simulink model "StartStop"  (R2021a)
settings: Solver=VariableStepAuto  StartTime=0.0  StopTime=10.0  RelTol=1e-3
undefined symbols (not defined in the file): cs_charge_deplete_bool, cs_electric_decel_spd, cs_electric_launch_spd_hi, cs_electric_launch_spd_lo, cs_hi_soc, cs_lo_soc, cs_off_trq_frac, cyc_mph, fc_map_spd, fc_max_trq, fc_on, fc_spd_scale, fc_trq_scale, fc_tstat, mc_map_spd, mc_max_trq, mc_overtrq_factor, mc_spd_scale, mc_trq_scale, tc_mc_to_fc_ratio, vc_fc_warm_tmp_frac, vc_idle_bool, vc_idle_spd, vc_key_on, vc_launch_spd
settings Model: Creator=thyag  LastModifiedBy=thyag

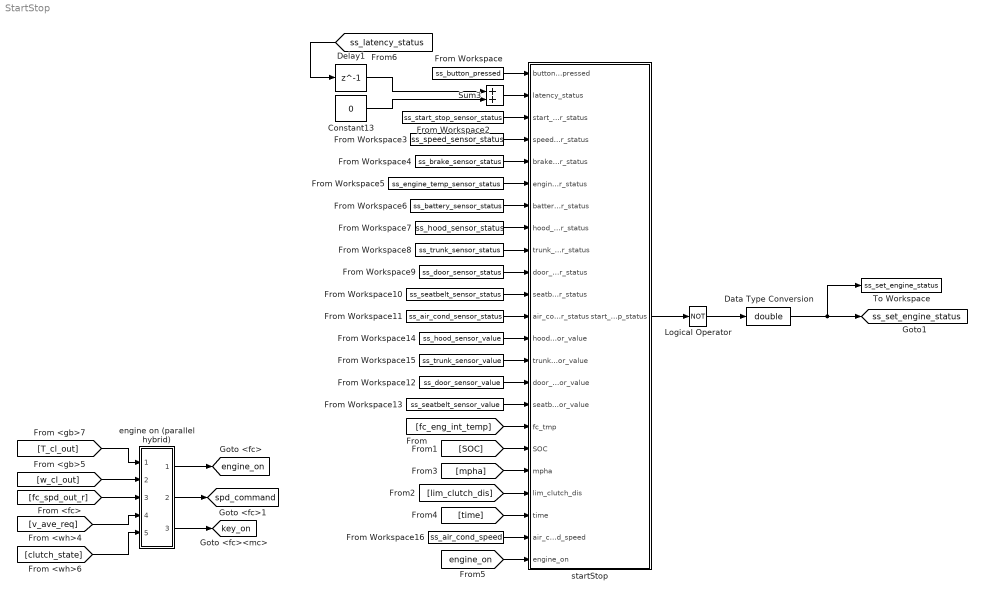
== system StartStop ==
  Constant13 : Constant  Value=0  OutDataTypeStr=fixdt(0,1,1,0)
  Data Type Conversion : DataTypeConversion  OutDataTypeStr=double
  Delay1 : Delay  DelayLength=1  InitialCondition=0
  From Workspace : FromWorkspace  VariableName=ss_button_pressed
  From Workspace10 : FromWorkspace  VariableName=ss_seatbelt_sensor_status
  From Workspace11 : FromWorkspace  VariableName=ss_air_cond_sensor_status
  From Workspace12 : FromWorkspace  VariableName=ss_door_sensor_value
  From Workspace13 : FromWorkspace  VariableName=ss_seatbelt_sensor_value
  From Workspace14 : FromWorkspace  VariableName=ss_hood_sensor_value
  From Workspace15 : FromWorkspace  VariableName=ss_trunk_sensor_value
  From Workspace16 : FromWorkspace  VariableName=ss_air_cond_speed
  From Workspace2 : FromWorkspace  VariableName=ss_start_stop_sensor_status
  From Workspace3 : FromWorkspace  VariableName=ss_speed_sensor_status
  From Workspace4 : FromWorkspace  VariableName=ss_brake_sensor_status
  From Workspace5 : FromWorkspace  VariableName=ss_engine_temp_sensor_status
  From Workspace6 : FromWorkspace  VariableName=ss_battery_sensor_status
  From Workspace7 : FromWorkspace  VariableName=ss_hood_sensor_status
  From Workspace8 : FromWorkspace  VariableName=ss_trunk_sensor_status
  From Workspace9 : FromWorkspace  VariableName=ss_door_sensor_status
  Logical Operator : Logic  Operator=NOT  AllPortsSameDT=off  OutDataTypeStr=fixdt(0,1,1,0)
  Sum3 : Sum  OutDataTypeStr=fixdt(0,1,1,0)
  To Workspace : ToWorkspace  VariableName=ss_set_engine_status  SampleTime=1
  engine on (parallel hybrid) : Subsystem
  startStop : Subsystem
  tag scope: engine_on=global, key_on=global, spd_command=global, ss_set_engine_status=global
  wires:
  engine on (parallel hybrid)/2(spd command (rad/s)) -> [spd_command]
  [v_ave_req] -> engine on (parallel hybrid)/4(v_ave_req)
  [ss_latency_status] -> Delay1/1
  [time] -> startStop/21(time)
  [engine_on] -> startStop/23(engine_on)
  Sum3/1 -> startStop/2(latency_status)
  Data Type Conversion/1 -> [ss_set_engine_status], To Workspace/1
  From Workspace13/1 -> startStop/16(seatbelt_sensor_value)
  From Workspace2/1 -> startStop/3(start_stop_sensor_status)
  Delay1/1 -> Sum3/1
  Constant13/1 -> Sum3/2
  From Workspace6/1 -> startStop/7(battery_sensor_status)
  From Workspace14/1 -> startStop/13(hood_sensor_value)
  From Workspace/1 -> startStop/1(button_pressed)
  [w_cl_out] -> engine on (parallel hybrid)/2(spd req'd out of clutch (N*m)1)
  [clutch_state] -> engine on (parallel hybrid)/5(clutch state)
  From Workspace8/1 -> startStop/9(trunk_sensor_status)
  startStop/1(start_stop_status) -> Logical Operator/1
  [T_cl_out] -> engine on (parallel hybrid)/1(trq req'd out of clutch (N*m))
  engine on (parallel hybrid)/3(key on) -> [key_on]
  [SOC] -> startStop/18(SOC)
  [fc_eng_int_temp] -> startStop/17(fc_tmp)
  [fc_spd_out_r] -> engine on (parallel hybrid)/3(fc_spd_out_r)
  From Workspace7/1 -> startStop/8(hood_sensor_status)
  Logical Operator/1 -> Data Type Conversion/1
  From Workspace15/1 -> startStop/14(trunk_sensor_value)
  From Workspace3/1 -> startStop/4(speed_sensor_status)
  From Workspace9/1 -> startStop/10(door_sensor_status)
  [mpha] -> startStop/19(mpha)
  engine on (parallel hybrid)/1(engine on) -> [engine_on]
  From Workspace12/1 -> startStop/15(door_sensor_value)
  From Workspace11/1 -> startStop/12(air_cond_sensor_status)
  From Workspace5/1 -> startStop/6(engine_temp_sensor_status)
  From Workspace10/1 -> startStop/11(seatbelt_sensor_status)
  [lim_clutch_dis] -> startStop/20(lim_clutch_dis)
  From Workspace16/1 -> startStop/22(air_cond_speed)
  From Workspace4/1 -> startStop/5(brake_sensor_status)

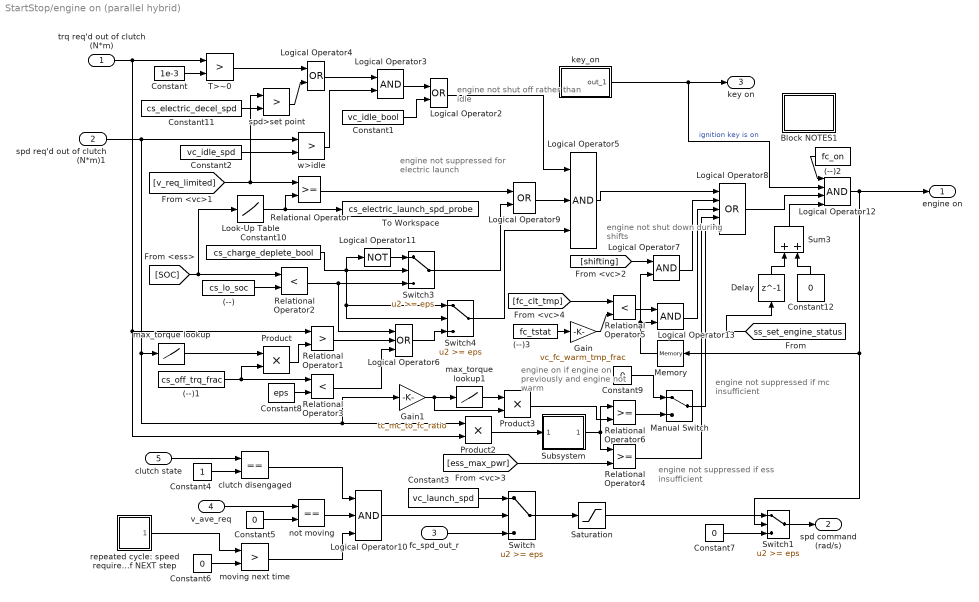
== system StartStop/engine on (parallel hybrid) ==
  note: engine not suppressed
      | if mc insufficient
  note: engine not shut
      | down during shifts
  note: engine on if engine on
      | previously and engine
      | not warm
  note: engine not shut off
      |  rather than idle
  note: engine not
      | suppressed for
      | electric launch
  note: engine not suppressed if
      | ess insufficient
  trq req'd out of clutch (N*m) : Inport
  spd req'd out of clutch (N*m)1 : Inport  Port=2
  fc_spd_out_r : Inport  Port=3
  v_ave_req : Inport  Port=4
  clutch state : Inport  Port=5
  (--) : Constant  Value=cs_lo_soc
  (--)1 : Constant  Value=cs_off_trq_frac
  (--)2 : Constant  Value=fc_on
  (--)3 : Constant  Value=fc_tstat
  Block NOTES1 : Subsystem
      mask Display: disp('Block\nNOTES')
  Constant : Constant  Value=1e-3
  Constant1 : Constant  Value=vc_idle_bool
  Constant10 : Constant  Value=cs_charge_deplete_bool
  Constant11 : Constant  Value=cs_electric_decel_spd
  Constant{5..7,9,12} (5 alike) : Constant  Value=0
  Constant2 : Constant  Value=vc_idle_spd
  Constant3 : Constant  Value=vc_launch_spd
  Constant4 : Constant
  Constant8 : Constant  Value=eps
  Delay : Delay  DelayLength=1  InitialCondition=1
  Gain : Gain  Gain=vc_fc_warm_tmp_frac  SaturateOnIntegerOverflow=on  OutDataTypeStr=Inherit: Same as input  ParamDataTypeStr=Inherit: Same as input
  Gain1 : Gain  Gain=tc_mc_to_fc_ratio  SaturateOnIntegerOverflow=on  OutDataTypeStr=Inherit: Same as input  ParamDataTypeStr=Inherit: Same as input
  Logical Operator10 : Logic  Inputs=3
  Logical Operator11 : Logic  Operator=NOT  Inputs=1
  Logical Operator12 : Logic  Inputs=4
  Logical Operator13 : Logic
  Logical Operator2 : Logic  Operator=OR
  Logical Operator3 : Logic
  Logical Operator4 : Logic  Operator=OR
  Logical Operator5 : Logic  Inputs=3
  Logical Operator6 : Logic  Operator=OR  Inputs=3
  Logical Operator7 : Logic
  Logical Operator8 : Logic  Operator=OR  Inputs=5
  Logical Operator9 : Logic  Operator=OR
  Look-Up Table : Lookup  InputValues=[cs_lo_soc cs_hi_soc cs_hi_soc+eps]  Table=[cs_electric_launch_spd_lo cs_electric_launch_spd_hi cs_electric_launch_spd_hi]  SaturateOnIntegerOverflow=on
  Manual Switch : ManualSwitch
  Memory : Memory  InitialCondition=cyc_mph(1,2)>0
  Product : Product  InputSameDT=on  RndMeth=Zero  SaturateOnIntegerOverflow=on  OutDataTypeStr=Inherit: Same as first input
  Product2 : Product  InputSameDT=on  RndMeth=Zero  SaturateOnIntegerOverflow=on  OutDataTypeStr=Inherit: Same as first input
  Product3 : Product  InputSameDT=on  RndMeth=Zero  SaturateOnIntegerOverflow=on  OutDataTypeStr=Inherit: Same as first input
  Relational Operator : RelationalOperator  RndMeth=Nearest  InputSameDT=on
  Relational Operator1 : RelationalOperator  Operator=>  RndMeth=Nearest  InputSameDT=on
  Relational Operator2 : RelationalOperator  Operator=<  RndMeth=Nearest  InputSameDT=on
  Relational Operator3 : RelationalOperator  Operator=<  RndMeth=Nearest  InputSameDT=on
  Relational Operator4 : RelationalOperator  RndMeth=Nearest  InputSameDT=on
  Relational Operator5 : RelationalOperator  Operator=<  RndMeth=Nearest  InputSameDT=on
  Relational Operator6 : RelationalOperator  RndMeth=Nearest  InputSameDT=on
  Saturation : Saturate  UpperLimit=max(fc_map_spd)*fc_spd_scale  LowerLimit=vc_idle_spd*vc_idle_bool
  Subsystem : Subsystem  mask(Running Average){n=3}
      mask prompts: n "Averaging Time Steps (#)"
      mask help: Running Average
      mask Help: Output is the average of the last (Averaging Time) seconds of input.
      mask Display: disp('Running\nAverage')
  Sum3 : Sum  Inputs=+|+
  Switch{,1,3..4} (4 alike) : Switch  Threshold=eps  SaturateOnIntegerOverflow=on  InputSameDT=on
  T>~0 : RelationalOperator  Operator=>  RndMeth=Nearest  InputSameDT=on
  To Workspace : ToWorkspace  VariableName=cs_electric_launch_spd_probe  SampleTime=-1
  clutch disengaged : RelationalOperator  Operator===  RndMeth=Nearest  InputSameDT=on
  key_on : Subsystem  mask(Repeating table){t=vc_key_on(:,1), y=vc_key_on(:,2)}
      mask prompts: t "Time values:"; y "Output values:"
      mask help:
      | Repeating table.
      | Enter values of time and output for first cycle.
      mask init:
      | period = max(t);
      mask Help: Repeats cycle given in table. Time values should be monotonically increasing.
  max_torque lookup : Lookup  InputValues=fc_map_spd*fc_spd_scale  Table=fc_max_trq*fc_trq_scale  SaturateOnIntegerOverflow=on
  max_torque lookup1 : Lookup  InputValues=mc_map_spd*mc_spd_scale  Table=mc_max_trq*mc_trq_scale*mc_overtrq_factor  SaturateOnIntegerOverflow=on
  moving next time : RelationalOperator  Operator=>  RndMeth=Nearest  InputSameDT=on
  not moving : RelationalOperator  Operator===  RndMeth=Nearest  InputSameDT=on
  repeated cycle: speed required at end of NEXT step : Subsystem  mask(Forward looking repeating table){t=cyc_mph(:,1), y=cyc_mph(:,2)}
      mask prompts: t "Time values:"; y "Output values:"
      mask help:
      | Forward looking repeating table.
      | Enter values of time and output for first cycle.
      mask init:
      | period = max(t);
      mask Help: Repeats cycle given in table with a one time step forward offset. Time values should be monotonically increasing.
  spd>set point : RelationalOperator  Operator=>  RndMeth=Nearest  InputSameDT=on
  w>idle : RelationalOperator  Operator=>  RndMeth=Nearest  InputSameDT=on
  engine on : Outport
  spd command (rad/s) : Outport  Port=2
  key on : Outport  Port=3
  wires:
  Subsystem/1(out_1) -> Relational Operator6/1, Relational Operator4/1
  Product3/1 -> Relational Operator6/2
  [ess_max_pwr] -> Relational Operator4/2
  [v_req_limited] -> spd>set point/1, Relational Operator/1
  T>~0/1 -> Logical Operator4/1
  Logical Operator4/1 -> Logical Operator3/1
  spd>set point/1 -> Logical Operator4/2
  Constant11/1 -> spd>set point/2
  spd req'd out of clutch (N*m)1/1 -> w>idle/1, Gain1/1, Product2/1, max_torque lookup/1
  w>idle/1 -> Logical Operator3/2
  Constant2/1 -> w>idle/2
  Constant9/1 -> Manual Switch/1
  Manual Switch/1 -> Logical Operator8/5
  Relational Operator6/1 -> Manual Switch/2
  Gain1/1 -> Product3/2, max_torque lookup1/1
  max_torque lookup1/1 -> Product3/1
  Relational Operator3/1 -> Logical Operator6/3
  Product2/1 -> Subsystem/1(in_1)
  Constant4/1 -> clutch disengaged/2
  clutch state/1 -> clutch disengaged/1
  Constant5/1 -> not moving/2
  v_ave_req/1 -> not moving/1
  not moving/1 -> Logical Operator10/2
  moving next time/1 -> Logical Operator10/3
  clutch disengaged/1 -> Logical Operator10/1
  Constant6/1 -> moving next time/2
  repeated cycle: speed required at end of NEXT step/1(out_1) -> moving next time/1
  Constant7/1 -> Switch1/3
  Switch1/1 -> spd command (rad/s)/1
  Saturation/1 -> Switch1/1
  fc_spd_out_r/1 -> Switch/3
  Logical Operator10/1 -> Switch/2
  Switch/1 -> Saturation/1
  Constant3/1 -> Switch/1
  Relational Operator4/1 -> Logical Operator8/4
  (--)/1 -> Relational Operator2/2
  [SOC] -> Look-Up Table/1, Relational Operator2/1
  Logical Operator11/1 -> Switch3/1
  Relational Operator2/1 -> Logical Operator6/1, Switch3/3
  Constant10/1 -> Logical Operator11/1, Switch3/2, Switch4/2, Switch4/1
  Look-Up Table/1 -> To Workspace/1, Relational Operator/2
  Relational Operator/1 -> Logical Operator9/1
  Switch4/1 -> Logical Operator5/3
  Logical Operator9/1 -> Logical Operator5/2
  Logical Operator2/1 -> Logical Operator5/1
  key_on/1(out_1) -> Logical Operator12/2, key on/1  "ignition key is on"
  Logical Operator8/1 -> Logical Operator12/3
  (--)3/1 -> Gain/1
  Gain/1 -> Relational Operator5/2
  Logical Operator13/1 -> Logical Operator8/3
  [fc_clt_tmp] -> Relational Operator5/1
  Relational Operator5/1 -> Logical Operator13/1
  Memory/1 -> Logical Operator13/2, Logical Operator7/2
  Relational Operator1/1 -> Logical Operator6/2
  Logical Operator5/1 -> Logical Operator8/1
  Logical Operator3/1 -> Logical Operator2/1
  Constant1/1 -> Logical Operator2/2
  trq req'd out of clutch (N*m)/1 -> Relational Operator1/1, Product2/2, T>~0/1
  Logical Operator7/1 -> Logical Operator8/2
  [shifting] -> Logical Operator7/1
  Constant/1 -> T>~0/2
  Switch3/1 -> Logical Operator9/2
  Logical Operator6/1 -> Switch4/3
  Constant8/1 -> Relational Operator3/2
  (--)1/1 -> Relational Operator3/1, Product/2
  Product/1 -> Relational Operator1/2
  max_torque lookup/1 -> Product/1
  (--)2/1 -> Logical Operator12/1
  Logical Operator12/1 -> engine on/1, Memory/1, Switch1/2
  [ss_set_engine_status] -> Delay/1
  Constant12/1 -> Sum3/2
  Sum3/1 -> Logical Operator12/4
  Delay/1 -> Sum3/1

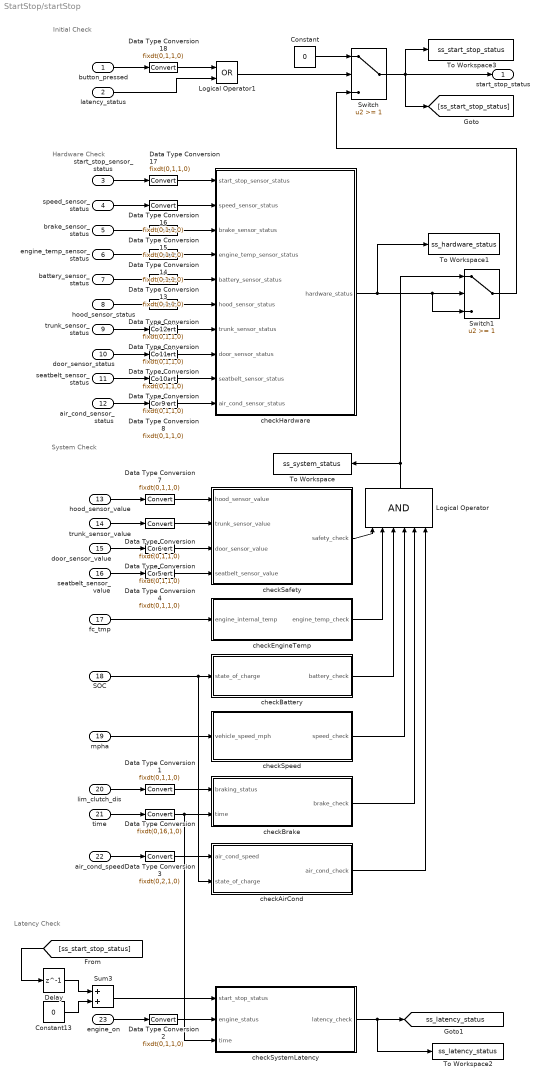
== system StartStop/startStop ==
  note: Initial Check
  note: Hardware Check
  note: Latency Check
  note: System Check
  button_pressed : Inport
  latency_status : Inport  Port=2
  start_stop_sensor_status : Inport  Port=3
  speed_sensor_status : Inport  Port=4
  brake_sensor_status : Inport  Port=5
  engine_temp_sensor_status : Inport  Port=6
  battery_sensor_status : Inport  Port=7
  hood_sensor_status : Inport  Port=8
  trunk_sensor_status : Inport  Port=9
  door_sensor_status : Inport  Port=10
  seatbelt_sensor_status : Inport  Port=11
  air_cond_sensor_status : Inport  Port=12
  hood_sensor_value : Inport  Port=13
  trunk_sensor_value : Inport  Port=14
  door_sensor_value : Inport  Port=15
  seatbelt_sensor_value : Inport  Port=16
  fc_tmp : Inport  Port=17
  SOC : Inport  Port=18
  mpha : Inport  Port=19
  lim_clutch_dis : Inport  Port=20
  time : Inport  Port=21
  air_cond_speed : Inport  Port=22
  engine_on : Inport  Port=23
  Constant : Constant  Value=0  OutDataTypeStr=fixdt(0,1,1,0)
  Constant13 : Constant  Value=0  OutDataTypeStr=fixdt(0,1,1,0)
  Data Type Conversion : DataTypeConversion  OutDataTypeStr=fixdt(0,16,1,0)
  Data Type Conversion{1..2,4..18} (17 alike) : DataTypeConversion  OutDataTypeStr=fixdt(0,1,1,0)
  Data Type Conversion3 : DataTypeConversion  OutDataTypeStr=fixdt(0,2,1,0)
  Delay : Delay  DelayLength=1  InitialCondition=0
  Logical Operator : Logic  Inputs=6  AllPortsSameDT=off  OutDataTypeStr=fixdt(0,1,1,0)
  Logical Operator1 : Logic  Operator=OR  AllPortsSameDT=off  OutDataTypeStr=fixdt(0,1,1,0)
  Sum3 : Sum  OutDataTypeStr=fixdt(0,1,1,0)
  Switch : Switch  Threshold=1  OutDataTypeStr=fixdt(0,1,1,0)
  Switch1 : Switch  Threshold=1  OutDataTypeStr=fixdt(0,1,1,0)
  To Workspace : ToWorkspace  VariableName=ss_system_status  SampleTime=-1
  To Workspace1 : ToWorkspace  VariableName=ss_hardware_status  SampleTime=-1
  To Workspace2 : ToWorkspace  VariableName=ss_latency_status  SampleTime=-1
  To Workspace3 : ToWorkspace  VariableName=ss_start_stop_status  SampleTime=-1
  checkAirCond : Subsystem
  checkBattery : Subsystem
  checkBrake : Subsystem
  checkEngineTemp : Subsystem
  checkHardware : Subsystem
  checkSafety : Subsystem
  checkSpeed : Subsystem
  checkSystemLatency : Subsystem
  start_stop_status : Outport
  tag scope: ss_latency_status=global
  wires:
  engine_temp_sensor_status/1 -> Data Type Conversion14/1
  speed_sensor_status/1 -> Data Type Conversion16/1
  Switch/1 -> [ss_start_stop_status], start_stop_status/1, To Workspace3/1
  trunk_sensor_status/1 -> Data Type Conversion11/1
  hood_sensor_status/1 -> Data Type Conversion12/1
  brake_sensor_status/1 -> Data Type Conversion15/1
  battery_sensor_status/1 -> Data Type Conversion13/1
  door_sensor_status/1 -> Data Type Conversion10/1
  seatbelt_sensor_status/1 -> Data Type Conversion9/1
  air_cond_sensor_status/1 -> Data Type Conversion8/1
  button_pressed/1 -> Data Type Conversion18/1
  latency_status/1 -> Logical Operator1/2
  Logical Operator1/1 -> Switch/2
  start_stop_sensor_status/1 -> Data Type Conversion17/1
  checkHardware/1(hardware_status) -> Switch1/2, Switch1/3, To Workspace1/1
  hood_sensor_value/1 -> Data Type Conversion7/1
  trunk_sensor_value/1 -> Data Type Conversion6/1
  door_sensor_value/1 -> Data Type Conversion5/1
  seatbelt_sensor_value/1 -> Data Type Conversion4/1
  fc_tmp/1 -> checkEngineTemp/1(engine_internal_temp)
  SOC/1 -> checkAirCond/2(state_of_charge), checkBattery/1(state_of_charge)
  mpha/1 -> checkSpeed/1(vehicle_speed_mph)
  air_cond_speed/1 -> Data Type Conversion3/1
  time/1 -> Data Type Conversion/1
  lim_clutch_dis/1 -> Data Type Conversion1/1
  checkSafety/1(safety_check) -> Logical Operator/1
  checkEngineTemp/1(engine_temp_check) -> Logical Operator/2
  checkBattery/1(battery_check) -> Logical Operator/3
  checkSpeed/1(speed_check) -> Logical Operator/4
  checkBrake/1(brake_check) -> Logical Operator/5
  checkAirCond/1(air_cond_check) -> Logical Operator/6
  Logical Operator/1 -> Switch1/1, To Workspace/1
  Constant/1 -> Switch/1
  Switch1/1 -> Switch/3
  engine_on/1 -> Data Type Conversion2/1
  checkSystemLatency/1(latency_check) -> [ss_latency_status], To Workspace2/1
  Sum3/1 -> checkSystemLatency/1(start_stop_status)
  [ss_start_stop_status] -> Delay/1
  Data Type Conversion/1 -> checkSystemLatency/3(time), checkBrake/2(time)
  Data Type Conversion1/1 -> checkBrake/1(braking_status)
  Data Type Conversion2/1 -> checkSystemLatency/2(engine_status)
  Data Type Conversion3/1 -> checkAirCond/1(air_cond_speed)
  Constant13/1 -> Sum3/2
  Delay/1 -> Sum3/1
  Data Type Conversion4/1 -> checkSafety/4(seatbelt_sensor_value)
  Data Type Conversion5/1 -> checkSafety/3(door_sensor_value)
  Data Type Conversion6/1 -> checkSafety/2(trunk_sensor_value)
  Data Type Conversion7/1 -> checkSafety/1(hood_sensor_value)
  Data Type Conversion8/1 -> checkHardware/10(air_cond_sensor_status)
  Data Type Conversion9/1 -> checkHardware/9(seatbelt_sensor_status)
  Data Type Conversion10/1 -> checkHardware/8(door_sensor_status)
  Data Type Conversion11/1 -> checkHardware/7(trunk_sensor_status)
  Data Type Conversion14/1 -> checkHardware/4(engine_temp_sensor_status)
  Data Type Conversion15/1 -> checkHardware/3(brake_sensor_status)
  Data Type Conversion13/1 -> checkHardware/5(battery_sensor_status)
  Data Type Conversion12/1 -> checkHardware/6(hood_sensor_status)
  Data Type Conversion16/1 -> checkHardware/2(speed_sensor_status)
  Data Type Conversion17/1 -> checkHardware/1(start_stop_sensor_status)
  Data Type Conversion18/1 -> Logical Operator1/1

== system StartStop/engine on (parallel hybrid)/Block NOTES1 ==
  note: This engine state computer keeps the engine on if:
      | [
      | 1) key is on, AND
      | 2) (trq is too high AND speed is too high for idle) OR engine is allowed to idle, AND
      | 3) vehicle speed >= cs_electric_launch_spd [ in m/s ], AND
      | 4) req'd trq > (cs_off_trq_frac * max_trq_at_spd) OR SOC<cs_lo_soc
      | ]
      | OR
      | [ engine was previously on AND the transmission is shifting ]
      |
      | The last condition is added to prevent the engine from unrealistically
      | shutting down for a second or two during a shift.

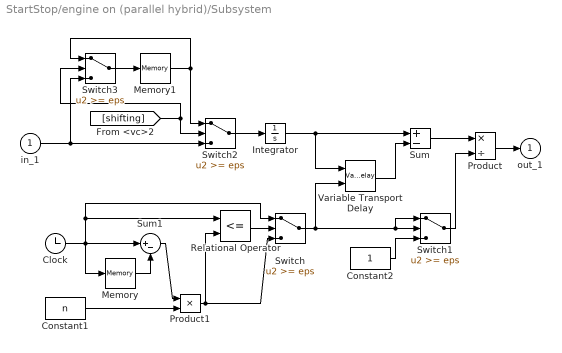
== system StartStop/engine on (parallel hybrid)/Subsystem ==
  in_1 : Inport
  Clock : Clock
  Constant1 : Constant  Value=n
  Constant2 : Constant
  Integrator : Integrator
  Memory : Memory  InitialCondition=-0.1
  Memory1 : Memory
  Product : Product  Inputs=*/  InputSameDT=on  RndMeth=Zero  SaturateOnIntegerOverflow=on  OutDataTypeStr=Inherit: Same as first input
  Product1 : Product  InputSameDT=on  RndMeth=Zero  SaturateOnIntegerOverflow=on  OutDataTypeStr=Inherit: Same as first input
  Relational Operator : RelationalOperator  Operator=<=  RndMeth=Nearest  InputSameDT=on
  Sum : Sum  Inputs=+-  InputSameDT=on  SaturateOnIntegerOverflow=on  OutDataTypeStr=Inherit: Same as first input
  Sum1 : Sum  Inputs=|+-  InputSameDT=on  SaturateOnIntegerOverflow=on  OutDataTypeStr=Inherit: Same as first input
  Switch{,1..3} (4 alike) : Switch  Threshold=eps  SaturateOnIntegerOverflow=on  InputSameDT=on
  Variable Transport Delay : VariableTransportDelay  MaximumDelay=n  ZeroDelay=on
  out_1 : Outport  InitialOutput=0
  wires:
  Product/1 -> out_1/1
  Sum/1 -> Product/1
  Variable Transport Delay/1 -> Sum/2
  Integrator/1 -> Variable Transport Delay/1, Sum/1
  Relational Operator/1 -> Switch/2
  Constant1/1 -> Product1/2
  Clock/1 -> Sum1/1, Memory/1, Relational Operator/1, Switch/1
  Memory/1 -> Sum1/2
  Sum1/1 -> Product1/1
  Product1/1 -> Relational Operator/2, Switch/3
  Switch/1 -> Variable Transport Delay/2, Switch1/2, Switch1/1
  Constant2/1 -> Switch1/3
  Switch1/1 -> Product/2
  Switch2/1 -> Integrator/1
  Switch3/1 -> Memory1/1
  in_1/1 -> Switch2/3, Switch3/3
  Memory1/1 -> Switch2/1, Switch3/1
  [shifting] -> Switch2/2, Switch3/2

== system StartStop/engine on (parallel hybrid)/key_on ==
  Clock : Clock
  Fcn1 : Fcn  Expr=rem(u[1],period)
  Look-Up Table : Lookup  InputValues=t  Table=y  SaturateOnIntegerOverflow=on
  out_1 : Outport  InitialOutput=0
  wires:
  Fcn1/1 -> Look-Up Table/1
  Clock/1 -> Fcn1/1
  Look-Up Table/1 -> out_1/1

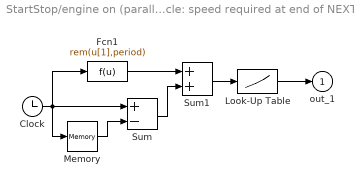
== system StartStop/engine on (parallel hybrid)/repeated cycle: speed required at end of NEXT step ==
  Clock : Clock
  Fcn1 : Fcn  Expr=rem(u[1],period)
  Look-Up Table : Lookup  InputValues=t  Table=y  SaturateOnIntegerOverflow=on
  Memory : Memory  InitialCondition=-0.1
  Sum : Sum  Inputs=+-  InputSameDT=on  SaturateOnIntegerOverflow=on  OutDataTypeStr=Inherit: Same as first input
  Sum1 : Sum  InputSameDT=on  SaturateOnIntegerOverflow=on  OutDataTypeStr=Inherit: Same as first input
  out_1 : Outport  InitialOutput=0
  wires:
  Sum1/1 -> Look-Up Table/1
  Look-Up Table/1 -> out_1/1
  Fcn1/1 -> Sum1/1
  Sum/1 -> Sum1/2
  Memory/1 -> Sum/2
  Clock/1 -> Fcn1/1, Memory/1, Sum/1

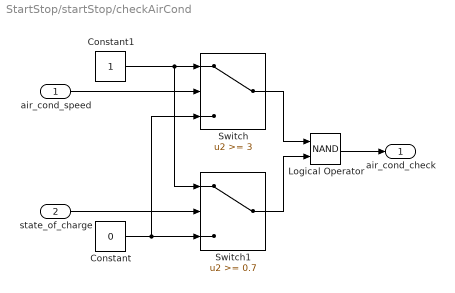
== system StartStop/startStop/checkAirCond ==
  air_cond_speed : Inport  OutDataTypeStr=fixdt(0,2,1,0)
  state_of_charge : Inport  Port=2
  Constant : Constant  Value=0  OutDataTypeStr=fixdt(0,1,1,0)
  Constant1 : Constant  OutDataTypeStr=fixdt(0,1,1,0)
  Logical Operator : Logic  Operator=NAND  AllPortsSameDT=off  OutDataTypeStr=fixdt(0,1,1,0)
  Switch : Switch  Threshold=3  OutDataTypeStr=fixdt(0,1,1,0)
  Switch1 : Switch  Threshold=0.7  OutDataTypeStr=fixdt(0,1,1,0)
  air_cond_check : Outport
  wires:
  Logical Operator/1 -> air_cond_check/1
  Switch/1 -> Logical Operator/1
  Switch1/1 -> Logical Operator/2
  state_of_charge/1 -> Switch1/2
  air_cond_speed/1 -> Switch/2
  Constant1/1 -> Switch1/1, Switch/1
  Constant/1 -> Switch/3, Switch1/3

== system StartStop/startStop/checkBattery ==
  state_of_charge : Inport
  Constant : Constant  Value=0  OutDataTypeStr=fixdt(0,1,1,0)
  Constant1 : Constant  OutDataTypeStr=fixdt(0,1,1,0)
  Switch : Switch  Criteria=u2 > Threshold  Threshold=0.5  OutDataTypeStr=fixdt(0,1,1,0)
  To Workspace : ToWorkspace  VariableName=ss_state_of_charge  SampleTime=-1
  battery_check : Outport
  wires:
  Switch/1 -> battery_check/1
  state_of_charge/1 -> Switch/2, To Workspace/1
  Constant/1 -> Switch/3
  Constant1/1 -> Switch/1

== system StartStop/startStop/checkBrake ==
  braking_status : Inport  OutDataTypeStr=fixdt(0,1,1,0)
  time : Inport  Port=2  OutDataTypeStr=fixdt(0,16,1,0)
  Switch : Switch  Threshold=1  OutDataTypeStr=fixdt(0,1,1,0)
  To Workspace : ToWorkspace  VariableName=ss_braking_status  SampleTime=-1
  checkBrakingElapsedTime : Subsystem
  brake_check : Outport
  wires:
  braking_status/1 -> checkBrakingElapsedTime/2(braking_status), To Workspace/1, Switch/3, Switch/2
  time/1 -> checkBrakingElapsedTime/1(time)
  checkBrakingElapsedTime/1(check_braking_elapsed_time) -> Switch/1
  Switch/1 -> brake_check/1

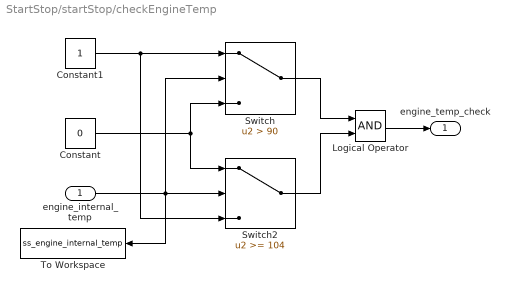
== system StartStop/startStop/checkEngineTemp ==
  engine_internal_temp : Inport
  Constant : Constant  Value=0  OutDataTypeStr=fixdt(0,1,1,0)
  Constant1 : Constant  OutDataTypeStr=fixdt(0,1,1,0)
  Logical Operator : Logic  AllPortsSameDT=off  OutDataTypeStr=fixdt(0,1,1,0)
  Switch : Switch  Criteria=u2 > Threshold  Threshold=90  OutDataTypeStr=fixdt(0,1,1,0)
  Switch2 : Switch  Threshold=104  OutDataTypeStr=fixdt(0,1,1,0)
  To Workspace : ToWorkspace  VariableName=ss_engine_internal_temp  SampleTime=-1
  engine_temp_check : Outport
  wires:
  Logical Operator/1 -> engine_temp_check/1
  engine_internal_temp/1 -> To Workspace/1, Switch/2, Switch2/2
  Constant/1 -> Switch2/1, Switch/3
  Constant1/1 -> Switch2/3, Switch/1
  Switch/1 -> Logical Operator/1
  Switch2/1 -> Logical Operator/2

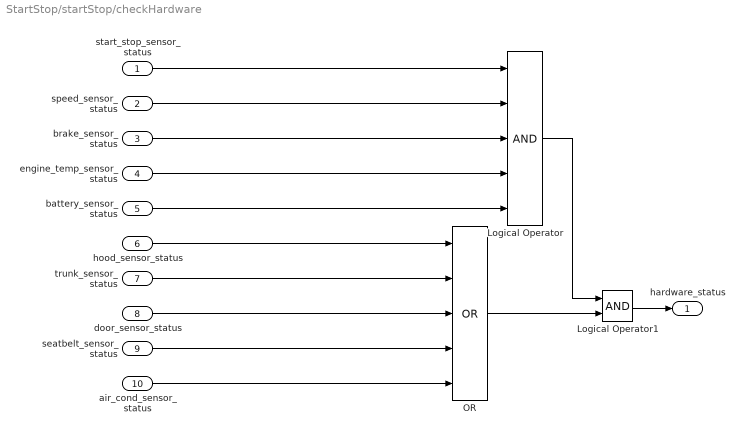
== system StartStop/startStop/checkHardware ==
  start_stop_sensor_status : Inport  OutDataTypeStr=fixdt(0,1,1,0)
  speed_sensor_status : Inport  Port=2  OutDataTypeStr=fixdt(0,1,1,0)
  brake_sensor_status : Inport  Port=3  OutDataTypeStr=fixdt(0,1,1,0)
  engine_temp_sensor_status : Inport  Port=4  OutDataTypeStr=fixdt(0,1,1,0)
  battery_sensor_status : Inport  Port=5  OutDataTypeStr=fixdt(0,1,1,0)
  hood_sensor_status : Inport  Port=6  OutDataTypeStr=fixdt(0,1,1,0)
  trunk_sensor_status : Inport  Port=7  OutDataTypeStr=fixdt(0,1,1,0)
  door_sensor_status : Inport  Port=8  OutDataTypeStr=fixdt(0,1,1,0)
  seatbelt_sensor_status : Inport  Port=9  OutDataTypeStr=fixdt(0,1,1,0)
  air_cond_sensor_status : Inport  Port=10  OutDataTypeStr=fixdt(0,1,1,0)
  Logical Operator : Logic  Inputs=5  AllPortsSameDT=off  OutDataTypeStr=fixdt(0,1,1,0)
  Logical Operator1 : Logic  AllPortsSameDT=off  OutDataTypeStr=fixdt(0,1,1,0)
  OR : Logic  Operator=OR  Inputs=5  AllPortsSameDT=off  OutDataTypeStr=fixdt(0,1,1,0)
  hardware_status : Outport
  wires:
  speed_sensor_status/1 -> Logical Operator/2
  brake_sensor_status/1 -> Logical Operator/3
  engine_temp_sensor_status/1 -> Logical Operator/4
  battery_sensor_status/1 -> Logical Operator/5
  hood_sensor_status/1 -> OR/1
  trunk_sensor_status/1 -> OR/2
  door_sensor_status/1 -> OR/3
  seatbelt_sensor_status/1 -> OR/4
  air_cond_sensor_status/1 -> OR/5
  Logical Operator1/1 -> hardware_status/1
  Logical Operator/1 -> Logical Operator1/1
  OR/1 -> Logical Operator1/2
  start_stop_sensor_status/1 -> Logical Operator/1

== system StartStop/startStop/checkSafety ==
  hood_sensor_value : Inport  OutDataTypeStr=fixdt(0,1,1,0)
  trunk_sensor_value : Inport  Port=2  OutDataTypeStr=fixdt(0,1,1,0)
  door_sensor_value : Inport  Port=3  OutDataTypeStr=fixdt(0,1,1,0)
  seatbelt_sensor_value : Inport  Port=4  OutDataTypeStr=fixdt(0,1,1,0)
  OR : Logic  Operator=OR  Inputs=4  AllPortsSameDT=off  OutDataTypeStr=fixdt(0,1,1,0)
  safety_check : Outport
  wires:
  hood_sensor_value/1 -> OR/1
  OR/1 -> safety_check/1
  trunk_sensor_value/1 -> OR/2
  door_sensor_value/1 -> OR/3
  seatbelt_sensor_value/1 -> OR/4

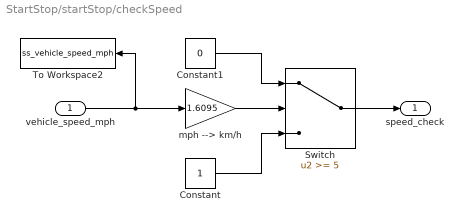
== system StartStop/startStop/checkSpeed ==
  vehicle_speed_mph : Inport
  Constant : Constant  OutDataTypeStr=fixdt(0,1,1,0)
  Constant1 : Constant  Value=0  OutDataTypeStr=fixdt(0,1,1,0)
  Switch : Switch  Threshold=5  OutDataTypeStr=fixdt(0,1,1,0)
  To Workspace2 : ToWorkspace  VariableName=ss_vehicle_speed_mph  SampleTime=-1
  mph --> km/h : Gain  Gain=1.6095
  speed_check : Outport
  wires:
  Switch/1 -> speed_check/1
  mph --> km/h/1 -> Switch/2
  vehicle_speed_mph/1 -> To Workspace2/1, mph --> km/h/1
  Constant1/1 -> Switch/1
  Constant/1 -> Switch/3

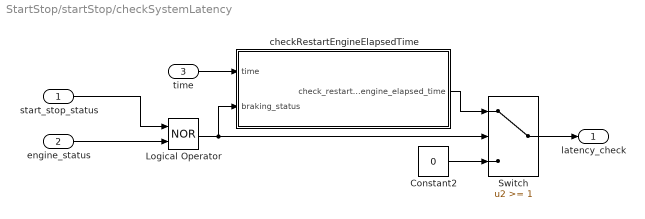
== system StartStop/startStop/checkSystemLatency ==
  start_stop_status : Inport
  engine_status : Inport  Port=2  OutDataTypeStr=fixdt(0,1,1,0)
  time : Inport  Port=3
  Constant2 : Constant  Value=0  OutDataTypeStr=fixdt(0,1,1,0)
  Logical Operator : Logic  Operator=NOR  AllPortsSameDT=off  OutDataTypeStr=fixdt(0,1,1,0)
  Switch : Switch  Threshold=1  OutDataTypeStr=fixdt(0,1,1,0)
  checkRestartEngineElapsedTime : Subsystem
  latency_check : Outport
  wires:
  Constant2/1 -> Switch/3
  Logical Operator/1 -> Switch/2, checkRestartEngineElapsedTime/2(braking_status)
  Switch/1 -> latency_check/1
  checkRestartEngineElapsedTime/1(check_restart_engine_elapsed_time) -> Switch/1
  time/1 -> checkRestartEngineElapsedTime/1(time)
  engine_status/1 -> Logical Operator/2
  start_stop_status/1 -> Logical Operator/1

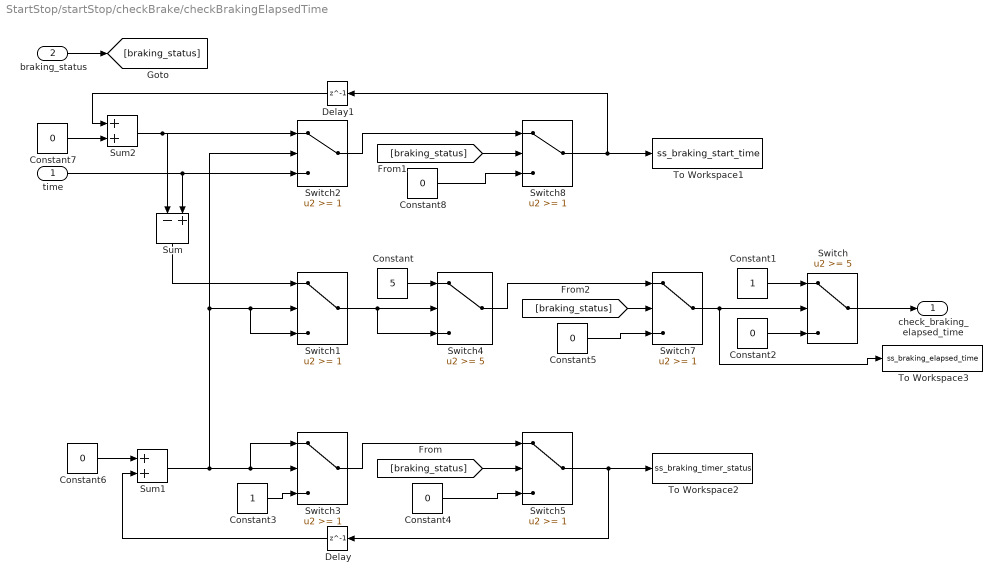
== system StartStop/startStop/checkBrake/checkBrakingElapsedTime ==
  time : Inport  OutDataTypeStr=fixdt(0,16,1,0)
  braking_status : Inport  Port=2  OutDataTypeStr=fixdt(0,1,1,0)
  Constant : Constant  Value=5  OutDataTypeStr=fixdt(0,3,1,0)
  Constant1 : Constant  OutDataTypeStr=fixdt(0,1,1,0)
  Constant{2,4..6,8} (5 alike) : Constant  Value=0  OutDataTypeStr=fixdt(0,1,1,0)
  Constant3 : Constant  OutDataTypeStr=fixdt(0,1,1,0)
  Constant7 : Constant  Value=0  OutDataTypeStr=fixdt(0,16,1,0)
  Delay : Delay  DelayLength=1  InitialCondition=0
  Delay1 : Delay  DelayLength=1  InitialCondition=0
  Sum : Sum  Inputs=-|+  OutDataTypeStr=fixdt(0,16,1,0)
  Sum1 : Sum  OutDataTypeStr=fixdt(0,1,1,0)
  Sum2 : Sum  OutDataTypeStr=fixdt(0,16,1,0)
  Switch : Switch  Threshold=5  OutDataTypeStr=fixdt(0,1,1,0)
  Switch{1..2,7..8} (4 alike) : Switch  Threshold=1  OutDataTypeStr=fixdt(0,16,1,0)
  Switch3 : Switch  Threshold=1  OutDataTypeStr=fixdt(0,1,1,0)
  Switch4 : Switch  Threshold=5
  Switch5 : Switch  Threshold=1  OutDataTypeStr=fixdt(0,1,1,0)
  To Workspace1 : ToWorkspace  VariableName=ss_braking_start_time  SampleTime=-1
  To Workspace2 : ToWorkspace  VariableName=ss_braking_timer_status  SampleTime=-1
  To Workspace3 : ToWorkspace  VariableName=ss_braking_elapsed_time  SampleTime=-1
  check_braking_elapsed_time : Outport
  wires:
  Sum/1 -> Switch1/1
  time/1 -> Sum/2, Switch2/3
  Sum2/1 -> Sum/1, Switch2/1
  Constant/1 -> Switch4/1
  Constant1/1 -> Switch/1
  Constant2/1 -> Switch/3
  Switch/1 -> check_braking_elapsed_time/1
  braking_status/1 -> [braking_status]
  [braking_status] -> Switch8/2
  [braking_status] -> Switch5/2
  Switch1/1 -> Switch4/2, Switch4/3
  Constant4/1 -> Switch5/3
  [braking_status] -> Switch7/2
  Constant5/1 -> Switch7/3
  Switch3/1 -> Switch5/1
  Switch4/1 -> Switch7/1
  Switch2/1 -> Switch8/1
  Constant3/1 -> Switch3/3
  Sum1/1 -> Switch2/2, Switch1/3, Switch1/2, Switch3/1, Switch3/2
  Switch8/1 -> Delay1/1, To Workspace1/1
  Switch7/1 -> To Workspace3/1, Switch/2
  Switch5/1 -> Delay/1, To Workspace2/1
  Constant6/1 -> Sum1/1
  Constant7/1 -> Sum2/2
  Constant8/1 -> Switch8/3
  Delay/1 -> Sum1/2
  Delay1/1 -> Sum2/1

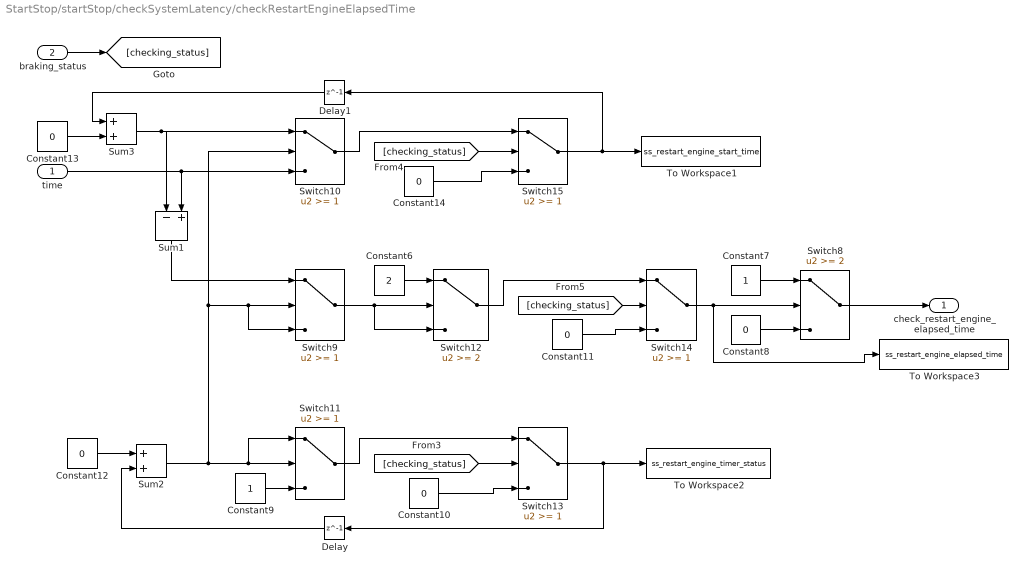
== system StartStop/startStop/checkSystemLatency/checkRestartEngineElapsedTime ==
  time : Inport  OutDataTypeStr=fixdt(0,16,1,0)
  braking_status : Inport  Port=2
  Constant{8,10..12,14} (5 alike) : Constant  Value=0  OutDataTypeStr=fixdt(0,1,1,0)
  Constant13 : Constant  Value=0  OutDataTypeStr=fixdt(0,16,1,0)
  Constant6 : Constant  Value=2  OutDataTypeStr=fixdt(0,2,1,0)
  Constant7 : Constant  OutDataTypeStr=fixdt(0,1,1,0)
  Constant9 : Constant  OutDataTypeStr=fixdt(0,1,1,0)
  Delay : Delay  DelayLength=1  InitialCondition=0
  Delay1 : Delay  DelayLength=1  InitialCondition=0
  Sum1 : Sum  Inputs=-|+  OutDataTypeStr=fixdt(0,16,1,0)
  Sum2 : Sum  OutDataTypeStr=fixdt(0,1,1,0)
  Sum3 : Sum  OutDataTypeStr=fixdt(0,16,1,0)
  Switch10 : Switch  Threshold=1  OutDataTypeStr=fixdt(0,16,1,0)
  Switch11 : Switch  Threshold=1  OutDataTypeStr=fixdt(0,1,1,0)
  Switch12 : Switch  Threshold=2
  Switch13 : Switch  Threshold=1  OutDataTypeStr=fixdt(0,1,1,0)
  Switch14 : Switch  Threshold=1
  Switch15 : Switch  Threshold=1  OutDataTypeStr=fixdt(0,16,1,0)
  Switch8 : Switch  Threshold=2  OutDataTypeStr=fixdt(0,1,1,0)
  Switch9 : Switch  Threshold=1
  To Workspace1 : ToWorkspace  VariableName=ss_restart_engine_start_time  SampleTime=-1
  To Workspace2 : ToWorkspace  VariableName=ss_restart_engine_timer_status  SampleTime=-1
  To Workspace3 : ToWorkspace  VariableName=ss_restart_engine_elapsed_time  SampleTime=-1
  check_restart_engine_elapsed_time : Outport
  wires:
  Constant14/1 -> Switch15/3
  Switch13/1 -> To Workspace2/1, Delay/1
  Switch11/1 -> Switch13/1
  Sum2/1 -> Switch10/2, Switch9/3, Switch9/2, Switch11/1, Switch11/2
  Delay1/1 -> Sum3/1
  Switch14/1 -> To Workspace3/1, Switch8/2
  Constant9/1 -> Switch11/3
  [checking_status] -> Switch14/2
  Switch8/1 -> check_restart_engine_elapsed_time/1
  Switch10/1 -> Switch15/1
  Sum1/1 -> Switch9/1
  Switch15/1 -> To Workspace1/1, Delay1/1
  time/1 -> Sum1/2, Switch10/3
  Constant11/1 -> Switch14/3
  Switch12/1 -> Switch14/1
  Constant10/1 -> Switch13/3
  Constant13/1 -> Sum3/2
  braking_status/1 -> [checking_status]
  Delay/1 -> Sum2/2
  [checking_status] -> Switch15/2
  [checking_status] -> Switch13/2
  Sum3/1 -> Sum1/1, Switch10/1
  Constant8/1 -> Switch8/3
  Constant7/1 -> Switch8/1
  Constant6/1 -> Switch12/1
  Switch9/1 -> Switch12/2, Switch12/3
  Constant12/1 -> Sum2/1
